simulink model "flexible_launcher_CL_filter"  (R2020b)
settings: Solver=ode23s  StartTime=0.0  StopTime=100  FixedStep=0.05  RelTol=1e-3  EnableMultiTasking=on
undefined symbols (not defined in the file or in its folder): afilt, ak, As, betafz, bfilt, bk, Bs, cfilt, ck, Cs, deltaW, dfilt, dhdx, dk, Ds, t0, thetac, ventonoff
settings Model: ExtModeAutoUpdateStatusClock=off  Creator=chiappa  LastModifiedBy=X000274
settings DataIOCC: LimitDataPoints=on  SaveFormat=Array  SignalLoggingSaveFormat=ModelDataLogs  ReturnWorkspaceOutputs=off  SignalLoggingName=sigsOut
settings OptimizationCC: BlockReduction=off  BooleanDataType=off
settings DebuggingCC: SaveWithParameterizedLinksMsg=none  UnderspecifiedInitializationDetection=Classic  MergeDetectMultiDrivingBlocksExec=none  SignalResolutionControl=TryResolveAllWithWarning  MultiTaskDSMMsg=warning  MultiTaskCondExecSysMsg=none  ArithmeticOperatorsInVariantConditions=warning
settings HardwareCC: ProdBitPerPointer=32  ProdBitPerSizeT=32  ProdBitPerPtrDiffT=32  ProdLargestAtomicFloat=None  ProdIntDivRoundTo=Undefined  ProdEndianess=Unspecified  ProdWordSize=32  ProdHWDeviceType=32-bit Generic  TargetUnknown=on
settings ModelReferenceCC: PropagateSignalLabelsOutOfModel=off
settings SFSimCC: SimUseLocalCustomCode=off  CustomCodeUndefinedFunction=UseInterfaceOnly
settings RTWCC: RTWUseLocalCustomCode=off
settings GRTTargetCC: TargetLangStandard=C89/C90 (ANSI)  CombineOutputUpdateFcns=off  GRTInterface=on
settings ConfigComp: CovMetricSettings=dw  CovSaveCumulativeToWorkspaceVar=on  CovSaveSingleToWorkspaceVar=on  CovExternalEMLEnable=off

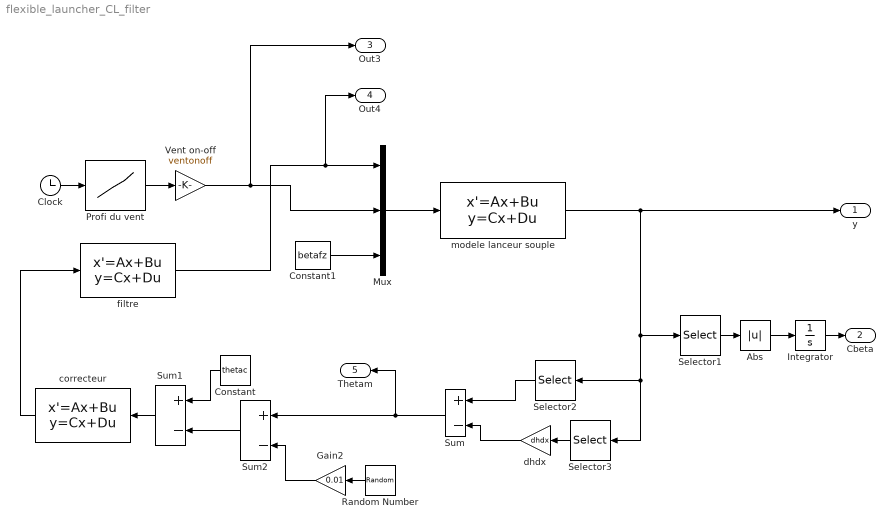
== system flexible_launcher_CL_filter ==
  Abs : Abs
  Clock : Clock
      settings: Decimation=100
  Constant : Constant  Value=thetac
  Constant1 : Constant  Value=betafz
  Gain2 : Gain  Gain=0.01  SaturateOnIntegerOverflow=on  OutDataTypeStr=Inherit: Same as input  ParamDataTypeStr=Inherit: Same as input
  Integrator : Integrator
  Mux : Mux  Inputs=3
  Profi du vent : Lookup  InputValues=t0  Table=deltaW  SaturateOnIntegerOverflow=on
  Random Number : RandomNumber  Variance=0.022*3.14/180  SampleTime=0.1
  Selector1 : Selector  InputPortWidth=8  IndexOptions=Index vector (dialog)  Indices=[4]  OutputSizes=1
  Selector2 : Selector  InputPortWidth=8  IndexOptions=Index vector (dialog)  Indices=[2]  OutputSizes=1
  Selector3 : Selector  InputPortWidth=8  IndexOptions=Index vector (dialog)  Indices=[7]  OutputSizes=1
  Sum : Sum  Inputs=+-  SaturateOnIntegerOverflow=on
  Sum1 : Sum  Inputs=+-  InputSameDT=on  SaturateOnIntegerOverflow=on  OutDataTypeStr=Inherit: Same as first input
  Sum2 : Sum  Inputs=+-  InputSameDT=on  SaturateOnIntegerOverflow=on  OutDataTypeStr=Inherit: Same as first input
  Vent on-off : Gain  Gain=ventonoff  SaturateOnIntegerOverflow=on  OutDataTypeStr=Inherit: Same as input  ParamDataTypeStr=Inherit: Same as input
  correcteur : StateSpace  A=ak  B=bk  C=ck  D=dk  InitialCondition=0
  dhdx : Gain  Gain=dhdx  SaturateOnIntegerOverflow=on  OutDataTypeStr=Inherit: Same as input  ParamDataTypeStr=Inherit: Same as input
  filtre : StateSpace  A=afilt  B=bfilt  C=cfilt  D=dfilt  InitialCondition=0
  modele lanceur souple : StateSpace  A=As  B=Bs  C=Cs  D=Ds  InitialCondition=0
  y : Outport  VectorParamsAs1DForOutWhenUnconnected=off
  Cbeta : Outport  Port=2  VectorParamsAs1DForOutWhenUnconnected=off
  Out3 : Outport  Port=3  VectorParamsAs1DForOutWhenUnconnected=off
  Out4 : Outport  Port=4  VectorParamsAs1DForOutWhenUnconnected=off
  Thetam : Outport  Port=5  VectorParamsAs1DForOutWhenUnconnected=off
  wires:
  Mux/1 -> modele lanceur souple/1
  modele lanceur souple/1 -> y/1, Selector1/1, Selector2/1, Selector3/1
  Selector1/1 -> Abs/1
  Abs/1 -> Integrator/1
  Integrator/1 -> Cbeta/1
  Selector2/1 -> Sum/1
  Selector3/1 -> dhdx/1
  Sum/1 -> Thetam/1, Sum2/1
  dhdx/1 -> Sum/2
  Clock/1 -> Profi du vent/1
  Profi du vent/1 -> Vent on-off/1
  Constant1/1 -> Mux/3
  Vent on-off/1 -> Out3/1, Mux/2
  Random Number/1 -> Gain2/1
  Gain2/1 -> Sum2/2
  filtre/1 -> Out4/1, Mux/1
  correcteur/1 -> filtre/1
  Sum2/1 -> Sum1/2
  Constant/1 -> Sum1/1
  Sum1/1 -> correcteur/1
